simulink model "FM"  (R2021b)
settings: Solver=VariableStepAuto  StartTime=0.0  StopTime=10  RelTol=1e-3
libraries: commanapbnd3 x1
settings Model: Creator=zhang  LastModifiedBy=zhang
settings SolverCC: AlgebraicLoopSolver=TrustRegion
settings DebuggingCC: SFMachineParentedDataDiag=warning

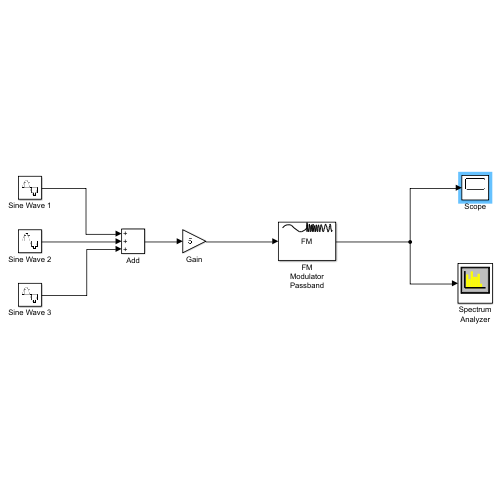
[thumbnail: Simulink's stored preview of the top-level diagram]
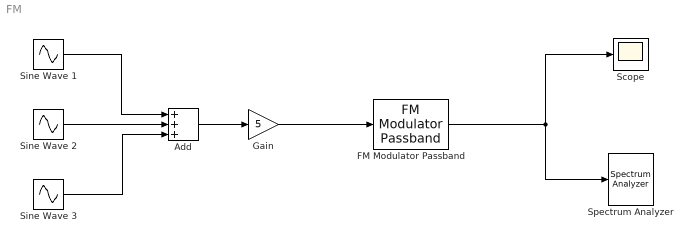
== system FM ==
  Add : Sum  Inputs=+++
  FM Modulator Passband : commanapbnd3/FM Modulator Passband  Fc=300  Ph=0  Kc=50
      settings: SourceProductBaseCode=CM
  Gain : Gain  Gain=5
  Scope : Scope
  Sine Wave 1 : Sin  Amplitude=0.3  Frequency=2*pi*10  SampleTime=1/3000
  Sine Wave 2 : Sin  Amplitude=0.2  Frequency=2*pi*20  Phase=pi/6  SampleTime=1/3000
  Sine Wave 3 : Sin  Amplitude=0.5  Frequency=2*pi*30  Phase=pi/3  SampleTime=1/3000
  Spectrum Analyzer : SpectrumAnalyzer
  wires:
  FM Modulator Passband/1 -> Spectrum Analyzer/1, Scope/1
  Sine Wave 2/1 -> Add/2
  Sine Wave 1/1 -> Add/1
  Sine Wave 3/1 -> Add/3
  Add/1 -> Gain/1
  Gain/1 -> FM Modulator Passband/1
